simulink model "Simulation_3D_LQR"  (R2016b)
settings: Solver=FixedStepAuto  StartTime=0.0  StopTime=10  FixedStep=0.001  RelTol=1e-3
values from neighbouring files (symbols this model uses):
  A = [zeros(3,3), g_LA, zeros(3,3) ... (first row only)    [RT_3D.m]
  B = [zeros(3,3); -I_K_inv; I_R_inv]    [RT_3D.m]
  F = lqr(reduced_SS.A, reduced_SS.B, Q, R)    [RT_3D.m]
  x_0 = ones(9,1)*0    [RT_3D.m]
undefined symbols (not defined in the file or in its folder): VK
settings Model: Creator=ich  LastModifiedBy=ich

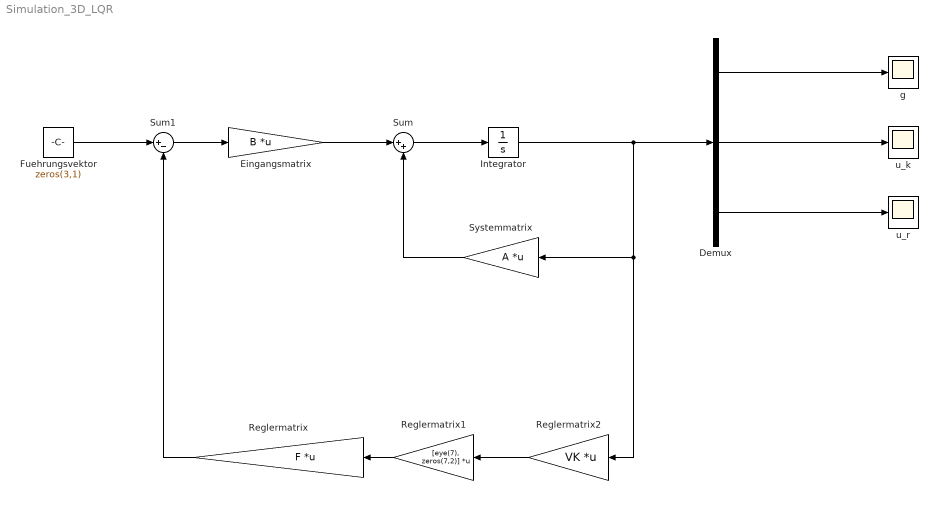
== system Simulation_3D_LQR ==
  Demux : Demux  Outputs=3
  Eingangsmatrix : Gain  Gain=B  Multiplication=Matrix(K*u) (u vector)
  Fuehrungsvektor : Constant  Value=zeros(3,1)
  Integrator : Integrator  InitialCondition=x_0
  Reglermatrix : Gain  Gain=F  Multiplication=Matrix(K*u) (u vector)
  Reglermatrix1 : Gain  Gain=[eye(7), zeros(7,2)]  Multiplication=Matrix(K*u) (u vector)
  Reglermatrix2 : Gain  Gain=VK  Multiplication=Matrix(K*u) (u vector)
  Sum : Sum  Inputs=|++  OutDataTypeStr=double
  Sum1 : Sum  Inputs=|+-
  Systemmatrix : Gain  Gain=A  Multiplication=Matrix(K*u) (u vector)
  g : Scope
  u_k : Scope
  u_r : Scope
  wires:
  Eingangsmatrix/1 -> Sum/1
  Systemmatrix/1 -> Sum/2
  Reglermatrix/1 -> Sum1/2
  Sum1/1 -> Eingangsmatrix/1
  Fuehrungsvektor/1 -> Sum1/1
  Sum/1 -> Integrator/1
  Integrator/1 -> Reglermatrix2/1, Systemmatrix/1, Demux/1
  Reglermatrix1/1 -> Reglermatrix/1
  Reglermatrix2/1 -> Reglermatrix1/1
  Demux/1 -> g/1
  Demux/2 -> u_k/1
  Demux/3 -> u_r/1
